simulink model "mrefrobotarm_modified_previous_y_previous_ref"  (R2018b)
settings: Solver=FixedStepAuto  StartTime=0.0  StopTime=60  RelTol=1e-3  AbsTol=1e-6
undefined symbols (not defined in the file or in its folder): sfunxy2
libraries: neural x301, simulink x1
(part 10 of 10)

== system mrefrobotarm_modified_previous_y_previous_ref/small_error/Layer 2/Delays 1 ==
  "p{2}" : Inport  PortDimensions=64
      mask Display: e = 0.06;c1 = [120 230 180]/255;c2 = ([120 230 180]+0)/(256+128);c3 = ([120 230 180]+128)/(256+128);patch([0 1 1 0],[0 0 1 1],c1);patch([0 1 1 1-e 1-e 0+e],[0 0 1 1-e 0+e 0+e],c2);patch([0 0 1 1-e 0+e 0+e],[0 1 1 1-e 1-e 0+e],c3);plot([0 1 1 0 0],[0 0 1 1 0]);
  mux : Mux  Inputs=1
      mask Display: e = 0.06;c1 = [120 150 230]/255;c2 = ([120 150 230]+0)/383;c3 = ([120 150 230]+128)/383;patch([0 1 1 0],[0 0 1 1],c1);patch([0 1 1 1-e 1-e 0+e],[0 0 1 1-e 0+e 0+e],c2);patch([0 0 1 1-e 0+e 0+e],[0 1 1 1-e 1-e 0+e],c3);plot([0 1 1 0 0],[0 0 1 1 0]);disp('Mux')
  "pd{2,1}" : Outport
      mask Display: e = 0.06;c1 = [120 230 180]/255;c2 = ([120 230 180]+0)/(256+128);c3 = ([120 230 180]+128)/(256+128);patch([0 1 1 0],[0 0 1 1],c1);patch([0 1 1 1-e 1-e 0+e],[0 0 1 1-e 0+e 0+e],c2);patch([0 0 1 1-e 0+e 0+e],[0 1 1 1-e 1-e 0+e],c3);plot([0 1 1 0 0],[0 0 1 1 0]);
  wires:
  "p{2}"/1 -> mux/1
  mux/1 -> "pd{2,1}"/1

== system mrefrobotarm_modified_previous_y_previous_ref/small_error/Layer 2/LW{2,1} ==
  "ad{2,1}" : Inport  PortDimensions=64
      mask Display: e = 0.06;c1 = [120 230 180]/255;c2 = ([120 230 180]+0)/(256+128);c3 = ([120 230 180]+128)/(256+128);patch([0 1 1 0],[0 0 1 1],c1);patch([0 1 1 1-e 1-e 0+e],[0 0 1 1-e 0+e 0+e],c2);patch([0 0 1 1-e 0+e 0+e],[0 1 1 1-e 1-e 0+e],c3);plot([0 1 1 0 0],[0 0 1 1 0]);
  "IW{2,1}(1,:)'" : Constant  Value=[-2.432056422256895444888868951238691806793212890625;0.0100380822801056680815268151718555600382387638092041015625;-0.00881928635249153679287470453118658042512834072113037109375;0.01603150923592765175751395645420416258275508880615234375;-0.1207510837780691181908565567937330342829227447509765625;0.444499867837198026077061285832314752042293548583984375;0.0685812208841292958449997740899561904370784759521484375;-0.0078652507082184568154570314391094143502414226531982421875;0.28537237524537040211924932009424082934856414794921875;0.319649219120275052130608628431218676269054412841796875;-0.248460759167887790255235813674516975879669189453125;0.0260047067229670463006652170179222594015300273895263671875;-0.0154576119356216838685025294353181379847228527069091796875;0.11961526310634827685586145662455237470567226409912109375;-0.09057560588763757802865939083858393132686614990234375;0.00761385824585609528869500906012035557068884372711181640625;0.0342736088456025156379070040202350355684757232666015625;-0.316084532035747989286988968160585500299930572509765625;-0.132128851048540163493072441269760020077228546142578125;-0.00870470025289365491316662115650615305639803409576416015625;0.005288189709423548982847318455924323643557727336883544921875;0.0168597088589711556483319299104550736956298351287841796875;0.004987064268464630988064723027264335541985929012298583984375;0.00962121920257344269422628002530473168008029460906982421875;0.00993019780836849712268854517560612293891608715057373046875;-0.040401077767249653216463656235646340064704418182373046875;0.00537110078625431704157922041531492141075432300567626953125;0.0244607043437967651422493275958913727663457393646240234375;-0.03215451369039921958314920402699499391019344329833984375;-0.1791695874091826234941748907658620737493038177490234375;0.0138555497359465172590997639190391055308282375335693359375;0.00508241101871751040086611084234391455538570880889892578125;0.0246713077469075565961720286622949060983955860137939453125;0.07283247848000092006248706866244901902973651885986328125;0.0237543328689119211116764773805698496289551258087158203125;0.06248637899898430714262786977997166104614734649658203125;0.1443238582260581159832923958674655295908451080322265625;-0.02724868663520964295887694106568233110010623931884765625;-0.0051694060515463415017567427867106744088232517242431640625;0.099369538513297939186230678387801162898540496826171875;-0.09836783955564017134509668949249316938221454620361328125;0.561885389335173623948094245861284434795379638671875;-0.0028850660115541108992343044548078978550620377063751220703125;0.036138786553751627017572189970451290719211101531982421875;-0.038930637620826692713027483705445774830877780914306640625;0.01399846512781122327695459972574099083431065082550048828125;0.0062092570377043874996214611883260658942162990570068359375;2.305316097006764319843341581872664391994476318359375;-0.007765227170624173190505157293728188960812985897064208984375;-0.03834582519997066507588812100948416627943515777587890625;-0.00486166535060293843184542339486142736859619617462158203125;-0.0031326623581803959665836867287680433946661651134490966796875;0.0253049226823349633630488852986673009581863880157470703125;-0.044554157526587305493404045364513876847922801971435546875;-0.039811627707193965319820705417441786266863346099853515625;0.29037743287937278768851001586881466209888458251953125;-0.0024393438826321024552601368640125656384043395519256591796875;0.726864176636829117938987110392190515995025634765625;-0.0091991907434141699517748946846040780656039714813232421875;-0.08749021728941898390363718363005318678915500640869140625;0.0079089487845599819315633993710434879176318645477294921875;0.0064178002501094934262315661044340231455862522125244140625;-0.0770159412457144532115904667080030776560306549072265625;0.0545713385970871822649996829568408429622650146484375]
      mask Display: e = 0.06;c1 = [120 150 230]/255;c2 = ([120 150 230]+0)/383;c3 = ([120 150 230]+128)/383;patch([0 1 1 0],[0 0 1 1],c1);patch([0 1 1 1-e 1-e 0+e],[0 0 1 1-e 0+e 0+e],c2);patch([0 0 1 1-e 0+e 0+e],[0 1 1 1-e 1-e 0+e],c3);plot([0 1 1 0 0],[0 0 1 1 0]);disp('weights');
  Mux : Mux  Inputs=1
      mask Display: e = 0.06;c1 = [120 150 230]/255;c2 = ([120 150 230]+0)/383;c3 = ([120 150 230]+128)/383;patch([0 1 1 0],[0 0 1 1],c1);patch([0 1 1 1-e 1-e 0+e],[0 0 1 1-e 0+e 0+e],c2);patch([0 0 1 1-e 0+e 0+e],[0 1 1 1-e 1-e 0+e],c3);plot([0 1 1 0 0],[0 0 1 1 0]);disp('Mux');
  dotprod1 : neural/Weight Functions/dotprod
  "lz{2,1}" : Outport
      mask Display: e = 0.06;c1 = [120 230 180]/255;c2 = ([120 230 180]+0)/(256+128);c3 = ([120 230 180]+128)/(256+128);patch([0 1 1 0],[0 0 1 1],c1);patch([0 1 1 1-e 1-e 0+e],[0 0 1 1-e 0+e 0+e],c2);patch([0 0 1 1-e 0+e 0+e],[0 1 1 1-e 1-e 0+e],c3);plot([0 1 1 0 0],[0 0 1 1 0]);
  wires:
  "IW{2,1}(1,:)'"/1 -> dotprod1/1
  "ad{2,1}"/1 -> dotprod1/2
  dotprod1/1 -> Mux/1
  Mux/1 -> "lz{2,1}"/1
